simulink library "visual_utility"  (R2020a)
settings: Solver=VariableStepAuto  StartTime=0.0  StopTime=10.0  RelTol=1e-3
settings Model: Creator=scastro  LastModifiedBy=rosha
settings DataIOCC: ReturnWorkspaceOutputs=off
settings DebuggingCC: PregeneratedLibrarySubsystemCodeDiagnostic=none  ArithmeticOperatorsInVariantConditions=warning
settings SFSimCC: SimUseLocalCustomCode=off  CustomCodeUndefinedFunction=UseInterfaceOnly
settings RTWCC: RTWUseLocalCustomCode=off

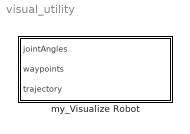
== system visual_utility ==
  my_Visualize Robot : MATLAB Function  InitFcn=clear visualizeRobot;  TreatAsAtomicUnit=on  mask(Visualize Robot){rbtName=gen3}
      mask prompts: rbtName "Rigid Body Tree Name"
      mask help: Displays a Rigid Body Tree, its waypoints, and end effector trajectory.

== matlab function visual_utility/my_Visualize Robot ==
  data: jointAngles input; waypoints input; trajectory input
function showRobot(jointAngles,waypoints,trajectory)
% Wrapper function that visualizes the robot in simulation.
       
    % Extract rigid body tree and end effector names from the block dialog
    coder.extrinsic('gcb');
    coder.extrinsic('get_param');
    persistent rbtName %eeName
    if isempty(rbtName)
       rbtName = get_param(gcb,'rbtName'); 
       %eeName = get_param(gcb,'eeName'); 
    end
    
    coder.extrinsic('visualizeRobot'); % Will be ignored for code generation
    visualizeRobot(rbtName,jointAngles,waypoints,trajectory);

end
